simulink model "pend_lin"  (R2018b)
settings: Solver=VariableStepAuto  StartTime=0.0  StopTime=20  RelTol=1e-10
values from neighbouring files (symbols this model uses):
  Jm = 3.1e-7    (= 3.1e-07)    [pend.m]
  Jp = 1774.274e-6    (= 0.001774274)    [pend.m]
  kd = 2    [pend.m]
  Kf = 7.44e-3    (= 0.00744)    [pend.m]
  kp = 20    [pend.m]
  La = 35e-6    (= 3.5e-05)    [pend.m]
  lb = 141.451e-3    (= 0.141451)    [pend.m]
  M = 879.5e-3    (= 0.8795)    [pend.m]
  m = 135.4e-3    (= 0.1354)    [pend.m]
  p1 = 0.0035    [cart_dumping.m]    (also in pend.m)
  p2 = 0.0058    [cart_dumping.m]    (also in pend.m)
  Ra = 3.92    [pend.m]
  Rg = 6.35e-3    (= 0.00635)    [pend.m]
  rt = 3.2067e-04    (= 0.00032067)    [pend.m]
  tet0 = pi/6    (= 0.523598775598)    [pend.m]
settings Model: Creator=lelli  LastModifiedBy=lelli
settings SFSimCC: SimUseLocalCustomCode=off
settings RTWCC: RTWUseLocalCustomCode=off

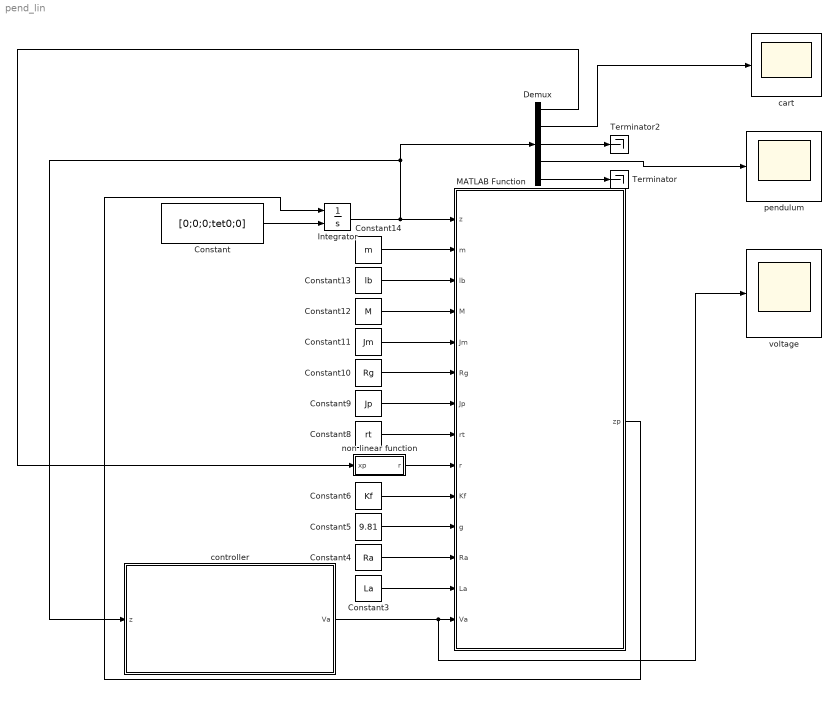
== system pend_lin ==
  Constant : Constant  Value=[0;0;0;tet0;0]
  Constant10 : Constant  Value=Rg
  Constant11 : Constant  Value=Jm
  Constant12 : Constant  Value=M
  Constant13 : Constant  Value=lb
  Constant14 : Constant  Value=m
  Constant3 : Constant  Value=La
  Constant4 : Constant  Value=Ra
  Constant5 : Constant  Value=9.81
  Constant6 : Constant  Value=Kf
  Constant8 : Constant  Value=rt
  Constant9 : Constant  Value=Jp
  Demux : Demux  Outputs=5
  Integrator : Integrator  InitialConditionSource=external
  MATLAB Function : MATLAB Function  TreatAsAtomicUnit=on
  Terminator : Terminator
  Terminator2 : Terminator
  cart : Scope
  controller : Subsystem
  non linear function : Subsystem
  pendulum : Scope
  voltage : Scope
  wires:
  Constant14/1 -> MATLAB Function/2(m)
  Constant13/1 -> MATLAB Function/3(lb)
  Constant11/1 -> MATLAB Function/5(Jm)
  Constant10/1 -> MATLAB Function/6(Rg)
  Constant9/1 -> MATLAB Function/7(Jp)
  Constant8/1 -> MATLAB Function/8(rt)
  Constant6/1 -> MATLAB Function/10(Kf)
  Constant5/1 -> MATLAB Function/11(g)
  Constant4/1 -> MATLAB Function/12(Ra)
  Constant3/1 -> MATLAB Function/13(La)
  Constant12/1 -> MATLAB Function/4(M)
  MATLAB Function/1(zp) -> Integrator/1
  Integrator/1 -> controller/1(z), Demux/1, MATLAB Function/1(z)
  Constant/1 -> Integrator/2
  Demux/4 -> pendulum/1
  Demux/2 -> cart/1
  Demux/1 -> non linear function/1(xp)
  Demux/3 -> Terminator2/1
  Demux/5 -> Terminator/1
  non linear function/1(r) -> MATLAB Function/9(r)
  controller/1(Va) -> voltage/1, MATLAB Function/14(Va)

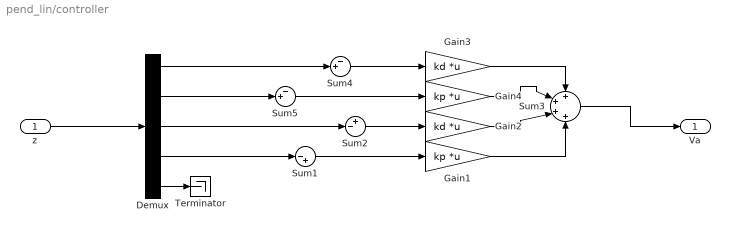
== system pend_lin/controller ==
  z : Inport
  Demux : Demux  Outputs=5
  Gain1 : Gain  Gain=kp  Multiplication=Matrix(K*u)
  Gain2 : Gain  Gain=kd  Multiplication=Matrix(K*u)
  Gain3 : Gain  Gain=kd  Multiplication=Matrix(K*u)
  Gain4 : Gain  Gain=kp  Multiplication=Matrix(K*u)
  Sum1 : Sum  Inputs=|-+
  Sum2 : Sum  Inputs=+-|
  Sum3 : Sum  Inputs=++++
  Sum4 : Sum  Inputs=-+|
  Sum5 : Sum  Inputs=-+|
  Terminator : Terminator
  Va : Outport
  wires:
  Sum3/1 -> Va/1
  z/1 -> Demux/1
  Sum2/1 -> Gain2/1
  Sum1/1 -> Gain1/1
  Gain1/1 -> Sum3/4
  Demux/5 -> Terminator/1
  Gain2/1 -> Sum3/3
  Demux/3 -> Sum2/2
  Demux/4 -> Sum1/1
  Gain4/1 -> Sum3/2
  Demux/2 -> Sum5/2
  Sum5/1 -> Gain4/1
  Gain3/1 -> Sum3/1
  Demux/1 -> Sum4/2
  Sum4/1 -> Gain3/1

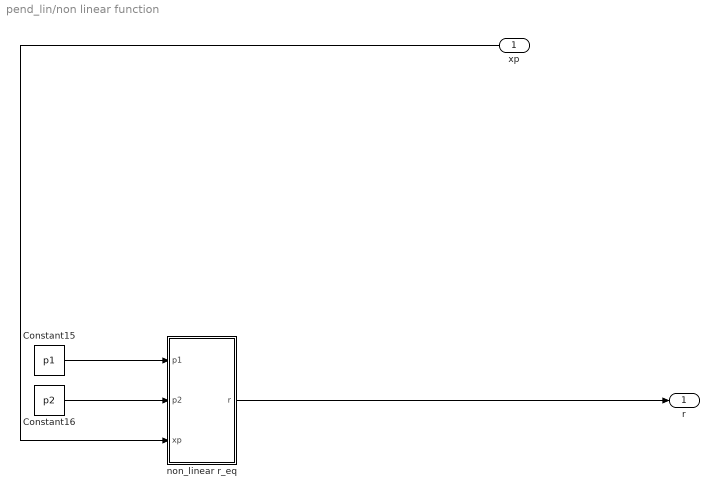
== system pend_lin/non linear function ==
  xp : Inport
  Constant15 : Constant  Value=p1
  Constant16 : Constant  Value=p2
  "non_linear r_eq " : MATLAB Function  TreatAsAtomicUnit=on
  r : Outport
  wires:
  Constant16/1 -> "non_linear r_eq "/2(p2)
  Constant15/1 -> "non_linear r_eq "/1(p1)
  "non_linear r_eq "/1(r) -> r/1
  xp/1 -> "non_linear r_eq "/3(xp)

== matlab function pend_lin/non linear function/non_linear r_eq  ==
  data: p1 input; r output; p2 input; xp input
function r  = r_eq(p1,p2,xp)
%non linear relationship between velocity and cart dumping
%p1 is the slope of linear approximation of force measured
%p2 is the intercept of linear approximation of force measured
%xp is the instantaneous velocity 
if xp>1e-10 || xp<-1e-10
    r=2*p2/pi*atan(100*xp)/xp + p1;
else
    r=2*p2/pi*100+p1;
end
end

== matlab function pend_lin/MATLAB Function ==
  data: z input; zp output; m input; lb input; M input; Jm input; Rg input; Jp input; rt input; r input; Kf input; g input; Ra input; La input; Va input
function zp = pend_lin_sys(z,m,lb,M,Jm,Rg,Jp,rt,r,Kf,g,Ra,La,Va)
%Va=kp*(-teta)+kd*(-tetap);

%z=[xp x tetap teta Ia];

M=[M + m + Jm/Rg^2 0 m*lb 0 0; 
   0 1 0 0 0; 
   m*lb 0 Jp+m*lb^2 0 0; 
   0 0 0 1 0;
   0 0 0 0 La]; %multipling Zp
N=[-r 0 0 0 -Kf/Rg;
    1 0 0 0 0;
    0 0 -rt -m*g*lb 0;
    0 0 1 0 0;
    Kf/Rg 0 0 0 -Ra]; %multipling Z
P=[0;
   0;
   0;
   0;
   1]; % multipling Va
A=(M\N);  B=M\P;
zp = A*z + B*Va;
